simulink model "ex6"  (Simulink 6.3)
settings: Solver=ode45  StartTime=0.0  StopTime=5000  RelTol=1e-3
values from neighbouring files (symbols this model uses):
  c1 = 2.94    [exp01e03.m]
  k1 = 338.6    [exp01e03.m]
  khw = 14732    [exp01e03.m]
  kpfA = 1 / Gps0    [exp01e03.m]
  kv = 0.005    [exp01e03.m]
  m1 = mc1 + mw1    (= 2.778)    [exp01e03.m]
settings Model: LastModifiedBy=aluno

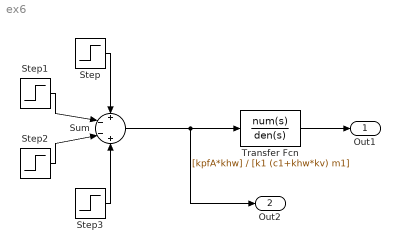
== system ex6 ==
  Step : Step  Time=1000  After=3000  SampleTime=0
  Step1 : Step  Time=2000  After=3000  SampleTime=0
  Step2 : Step  Time=3000  After=3000  SampleTime=0
  Step3 : Step  Time=4000  After=3000  SampleTime=0
  Sum : Sum  Inputs=+--+
  Transfer Fcn : TransferFcn  Numerator=[kpfA*khw]  Denominator=[k1 (c1+khw*kv) m1]
  Out1 : Outport
  Out2 : Outport  Port=2
  wires:
  Step/1 -> Sum/1
  Step1/1 -> Sum/2
  Transfer Fcn/1 -> Out1/1
  Step3/1 -> Sum/4
  Step2/1 -> Sum/3
  Sum/1 -> Transfer Fcn/1, Out2/1
